simulink model "digital10"  (R2024a)
settings: Solver=VariableStepAuto  StartTime=0.0  StopTime=10.0  RelTol=1e-3
settings Model: Creator=tusha  LastModifiedBy=tusha

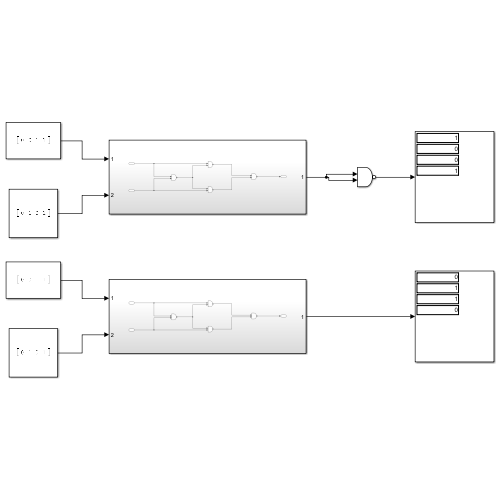
[thumbnail: Simulink's stored preview of the top-level diagram]
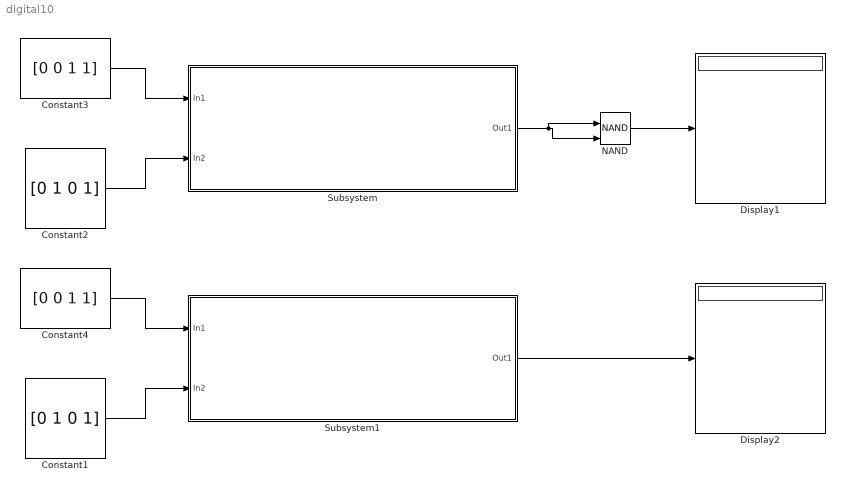
== system digital10 ==
  Constant1 : Constant  Value=[0 1 0 1]
  Constant2 : Constant  Value=[0 1 0 1]
  Constant3 : Constant  Value=[0 0 1 1]
  Constant4 : Constant  Value=[0 0 1 1]
  Display1 : Display
  Display2 : Display
  NAND : Logic  Operator=NAND  IconShape=distinctive  AllPortsSameDT=off  OutDataTypeStr=boolean
  Subsystem : Subsystem
  Subsystem1 : Subsystem
  wires:
  Constant3/1 -> Subsystem/1(In1)
  Constant2/1 -> Subsystem/2(In2)
  Subsystem/1(Out1) -> NAND/2, NAND/1
  NAND/1 -> Display1/1
  Subsystem1/1(Out1) -> Display2/1
  Constant1/1 -> Subsystem1/2(In2)
  Constant4/1 -> Subsystem1/1(In1)

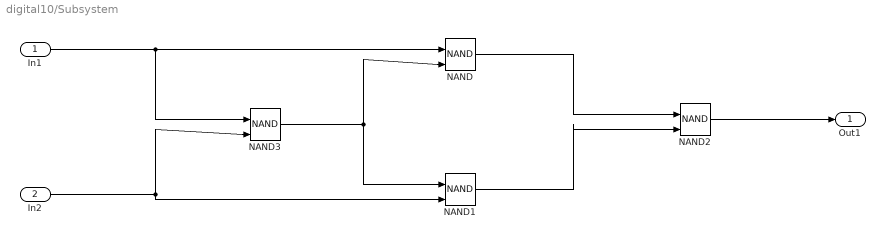
== system digital10/Subsystem ==
  In1 : Inport
  In2 : Inport  Port=2
  NAND{,1..3} (4 alike) : Logic  Operator=NAND  IconShape=distinctive  AllPortsSameDT=off  OutDataTypeStr=boolean
  Out1 : Outport
  wires:
  NAND1/1 -> NAND2/2
  NAND/1 -> NAND2/1
  In1/1 -> NAND3/1, NAND/1
  NAND3/1 -> NAND/2, NAND1/1
  In2/1 -> NAND3/2, NAND1/2
  NAND2/1 -> Out1/1

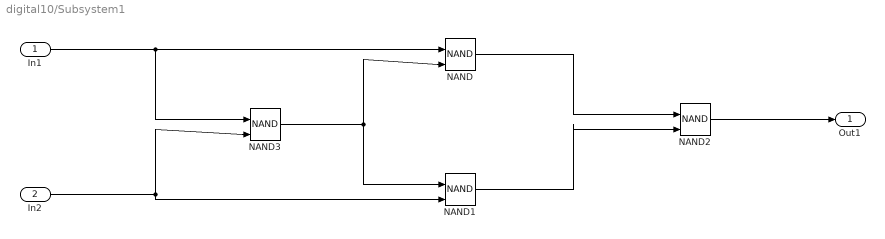
== system digital10/Subsystem1 ==
  In1 : Inport
  In2 : Inport  Port=2
  NAND{,1..3} (4 alike) : Logic  Operator=NAND  IconShape=distinctive  AllPortsSameDT=off  OutDataTypeStr=boolean
  Out1 : Outport
  wires:
  NAND1/1 -> NAND2/2
  NAND/1 -> NAND2/1
  In1/1 -> NAND3/1, NAND/1
  NAND3/1 -> NAND/2, NAND1/1
  In2/1 -> NAND3/2, NAND1/2
  NAND2/1 -> Out1/1
